simulink model "lab3_sim"  (R2019b)
settings: Solver=FixedStepAuto  StartTime=0.0  StopTime=10  FixedStep=1e-4  RelTol=1e-3
values from neighbouring files (symbols this model uses):
  A = [0, 1, 0, 0;-ks/ms, -T/ms, ks/ms, 0;0, 0, 0, 1;ks/mp, T/mp, -(ks + kp)/mp, -cp/mp]    [lab3_Task_4.m]    (also in lab3_Task_5.m = [0, 1, 0, 0; lab3_Task_5_old.m = [0, 1, 0, 0)
  B = [0, 0; 0, 0; 0, 0; kp/mp, cp/mp]    [lab3_Task_4.m]    (also in lab3_Task_5.m = [0,0,0,0; lab3_Task_5_old.m = [0,0,0,0)
undefined symbols (not defined in the file or in its folder): sigbuilder_block
settings Model: Creator=Hp  LastModifiedBy=Hp

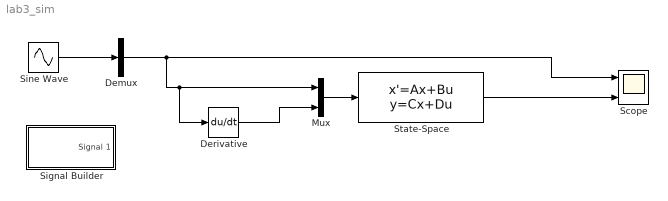
== system lab3_sim ==
  Demux : Demux  Outputs=1
  Derivative : Derivative
  Mux : Mux  Inputs=2
  Scope : Scope  NumInputPorts=3
  Signal Builder : Subsystem  Tag=STV Subsys  LoadFcn=sigbuilder_block('load');  StartFcn=sigbuilder_block('start');  StopFcn=sigbuilder_block('stop');  ClipboardFcn=sigbuilder_block('clipboard');  mask(Sigbuilder block){tuvar=[0:10]}
      mask help: Simulink:masks:SigbuilderBlock_MD
      mask init:
      | if ~strcmp(get_param(bdroot(gcbh),'SimulationStatus'),'stopped') tuvar = sigbuilder_block('maskInit'); end
      settings: CopyFcn=sigbuilder_block('copy');  DeleteFcn=sigbuilder_block('delete');  ModelCloseFcn=sigbuilder_block('modelClose');  PreSaveFcn=sigbuilder_block('preSave');  PauseFcn=sigbuilder_block('pause');  ContinueFcn=sigbuilder_block('continue');  NameChangeFcn=sigbuilder_block('namechange');  OpenFcn=sigbuilder_block('open',[404 117.5 550.5 362.5 ]);  CloseFcn=sigbuilder_block('close');
      mask Display: plot(0, 0, 100, 100,[2, 2, 32, 32, 2], [68, 8, 8, 68, 68],[32, 2], [38, 38], [32, 19, 2],[53, 60, 44], [32, 17, 17, 2],[16, 16, 31, 31]);txt = getActiveGroup(gcbh);text(2, 100, txt,'verticalAlignment', 'top');
  Sine Wave : Sin  Amplitude=0.05  Frequency=25  SampleTime=0
  State-Space : StateSpace  A=A  B=B  C=[1 0 0 0]  D=[0 0]  InitialCondition=0  ContinuousStateAttributes={'zs','zs_dot','zp','zp_dot'}
  wires:
  Derivative/1 -> Mux/2
  Mux/1 -> State-Space/1
  State-Space/1 -> Scope/3
  Sine Wave/1 -> Demux/1
  Demux/1 -> Scope/1, Derivative/1, Mux/1

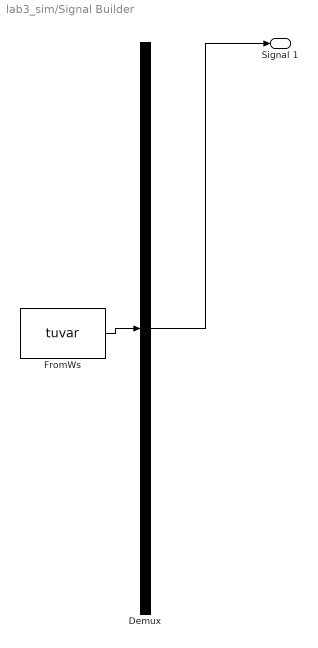
== system lab3_sim/Signal Builder ==
  Demux : Demux  Tag=STV Demux  Outputs=1
  FromWs : FromWorkspace  Tag=STV FromWs  VariableName=tuvar  SampleTime=0
      SigBuilderData=|
      | common.afterFinalStr = 'Extrapolate'
      | common.sampleTime = 0
      | dataSet.timeRange = [0 60]
      | dataSet.name = 'Group 1'
      | sbobj.Groups.Name = 'Group 1'
      | sbobj.Groups.Signals.Name = 'Signal 1'
      | sbobj.Groups.Signals.XData = [0 4 4 24 24 60]
      | sbobj.Groups.Signals.YData = [0 0 0.05 0.05 0 0]
      | sbobj.Groups.TimeRange = [0 60]
  Signal 1 : Outport  Tag=STV Outport
  wires:
  Demux/1 -> Signal 1/1
  FromWs/1 -> Demux/1
